simulink model "FrictionIdentification"  (Simulink 8.6)
settings: Solver=FixedStepDiscrete  StartTime=0.0  StopTime=120  FixedStep=robot.Ts  RelTol=1e-3
libraries: WBToolboxLibrary x15
settings Model: Creator=Raffaello  LastModifiedBy=DanielePucci
settings DataIOCC: LimitDataPoints=off  SignalLoggingSaveFormat=Dataset  OutputSaveName=out
settings OptimizationCC: ExpressionDepthLimit=128
settings DebuggingCC: InheritedTsInSrcMsg=none  FcnCallInpInsideContextMsg=EnableAllAsError
settings GRTTargetCC: CombineOutputUpdateFcns=on  GRTInterface=off
settings ConfigComp: CovSFcnEnable=off

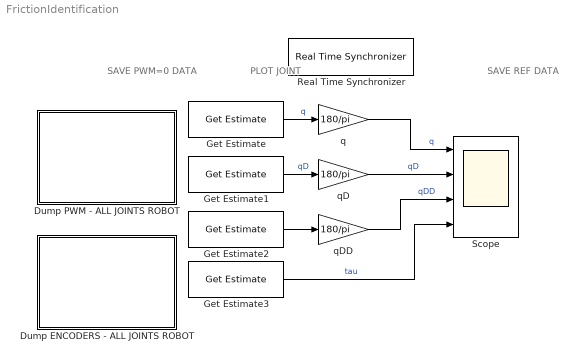
== system FrictionIdentification ==
  note: SAVE
      | PWM=0
      | DATA
  note: SAVE
      | REF DATA
  note: PLOT
      | JOINT
  Dump ENCODERS - ALL JOINTS ROBOT : Subsystem  mask{output='getMotorEncoderSpeeds'}
      mask prompts: output "Output port"
      mask Display:
      | color('red'); plot([10 20 30 40], [10 20 10 15]);
      | color('blue'); plot([10 20 30 40], [15 10 20 12]);
      | color('green'); plot([10 20 30 40], [13 16 12 18]);
  Dump PWM - ALL JOINTS ROBOT : Subsystem  mask{output='getOutputs'}
      mask prompts: output "Output port"
      mask Display:
      | color('red'); plot([10 20 30 40], [10 20 10 15]);
      | color('blue'); plot([10 20 30 40], [15 10 20 12]);
      | color('green'); plot([10 20 30 40], [13 16 12 18]);
  Get Estimate : WBToolboxLibrary/wholeBodyStates/Get Estimate  estimateType=Joints Position  robotName=WBT_robotName  localName=WBT_modelName  wbiFile=WBT_wbiFilename  wbiList=WBT_wbiList
  Get Estimate1 : WBToolboxLibrary/wholeBodyStates/Get Estimate  estimateType=Joints Velocity  robotName=WBT_robotName  localName=WBT_modelName  wbiFile=WBT_wbiFilename  wbiList=WBT_wbiList
  Get Estimate2 : WBToolboxLibrary/wholeBodyStates/Get Estimate  estimateType=Joints Acceleration  robotName=WBT_robotName  localName=WBT_modelName  wbiFile=WBT_wbiFilename  wbiList=WBT_wbiList
  Get Estimate3 : WBToolboxLibrary/wholeBodyStates/Get Estimate  estimateType=Joints Torque  robotName=WBT_robotName  localName=WBT_modelName  wbiFile=WBT_wbiFilename  wbiList=WBT_wbiList
  Real Time Synchronizer : WBToolboxLibrary/Utilities/Real Time Synchronizer  period=robot.Ts
  Scope : Scope  NumInputPorts=4
  q : Gain  Gain=180/pi
  qD : Gain  Gain=180/pi
  qDD : Gain  Gain=180/pi
  wires:
  Get Estimate/1 -> q/1  "q"
  Get Estimate1/1 -> qD/1  "qD"
  Get Estimate3/1 -> Scope/4  "tau"
  q/1 -> Scope/1  "q"
  qD/1 -> Scope/2  "qD"
  Get Estimate2/1 -> qDD/1
  qDD/1 -> Scope/3  "qDD"

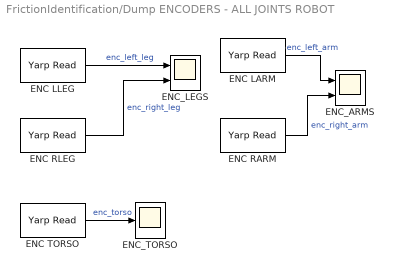
== system FrictionIdentification/Dump ENCODERS - ALL JOINTS ROBOT ==
  ENC LARM : WBToolboxLibrary/Utilities/Yarp Read  portName=PORTS.ENCODERS.LARM  signalSize=5  blocking=off  timestamp=off  autoconnect=on  errorOnConnection=off
  ENC LLEG : WBToolboxLibrary/Utilities/Yarp Read  portName=PORTS.ENCODERS.LLEG  signalSize=6  blocking=off  timestamp=off  autoconnect=on  errorOnConnection=off
  ENC RARM : WBToolboxLibrary/Utilities/Yarp Read  portName=PORTS.ENCODERS.RARM  signalSize=5  blocking=off  timestamp=off  autoconnect=on  errorOnConnection=off
  ENC RLEG : WBToolboxLibrary/Utilities/Yarp Read  portName=PORTS.ENCODERS.RLEG  signalSize=6  blocking=off  timestamp=off  autoconnect=on  errorOnConnection=off
  ENC TORSO : WBToolboxLibrary/Utilities/Yarp Read  portName=PORTS.ENCODERS.RARM  signalSize=3  blocking=off  timestamp=off  autoconnect=on  errorOnConnection=off
  ENC_ARMS : Scope  NumInputPorts=2
  ENC_LEGS : Scope  NumInputPorts=2
  ENC_TORSO : Scope
  wires:
  ENC LARM/1 -> ENC_ARMS/1  "enc_left_arm"
  ENC RARM/1 -> ENC_ARMS/2  "enc_right_arm"
  ENC TORSO/1 -> ENC_TORSO/1  "enc_torso"
  ENC RLEG/1 -> ENC_LEGS/2  "enc_right_leg"
  ENC LLEG/1 -> ENC_LEGS/1  "enc_left_leg"

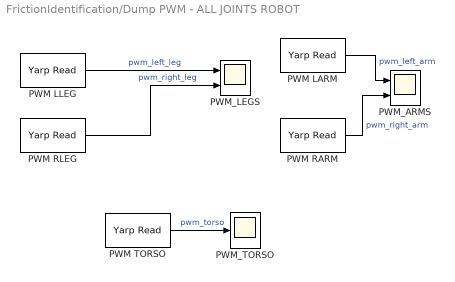
== system FrictionIdentification/Dump PWM - ALL JOINTS ROBOT ==
  PWM LARM : WBToolboxLibrary/Utilities/Yarp Read  portName=PORTS.PWM.LARM  signalSize=5  blocking=off  timestamp=off  autoconnect=on  errorOnConnection=off
  PWM LLEG : WBToolboxLibrary/Utilities/Yarp Read  portName=PORTS.PWM.LLEG  signalSize=6  blocking=off  timestamp=off  autoconnect=on  errorOnConnection=off
  PWM RARM : WBToolboxLibrary/Utilities/Yarp Read  portName=PORTS.PWM.RARM  signalSize=5  blocking=off  timestamp=off  autoconnect=on  errorOnConnection=off
  PWM RLEG : WBToolboxLibrary/Utilities/Yarp Read  portName=PORTS.PWM.RLEG  signalSize=6  blocking=off  timestamp=off  autoconnect=on  errorOnConnection=off
  PWM TORSO : WBToolboxLibrary/Utilities/Yarp Read  portName=PORTS.PWM.TORSO  signalSize=3  blocking=off  timestamp=off  autoconnect=on  errorOnConnection=off
  PWM_ARMS : Scope  NumInputPorts=2
  PWM_LEGS : Scope  NumInputPorts=2
  PWM_TORSO : Scope
  wires:
  PWM LARM/1 -> PWM_ARMS/1  "pwm_left_arm"
  PWM RARM/1 -> PWM_ARMS/2  "pwm_right_arm"
  PWM TORSO/1 -> PWM_TORSO/1  "pwm_torso"
  PWM LLEG/1 -> PWM_LEGS/1  "pwm_left_leg"
  PWM RLEG/1 -> PWM_LEGS/2  "pwm_right_leg"
